simulink model "SimuRun_Day1_Val"  (R2020a)
settings: Solver=FixedStepAuto  StartTime=86400*0+360*60  StopTime=86400*0+1200*60  FixedStep=60  RelTol=1e-6
settings Model: Creator=zhelu  LastModifiedBy=yl3328

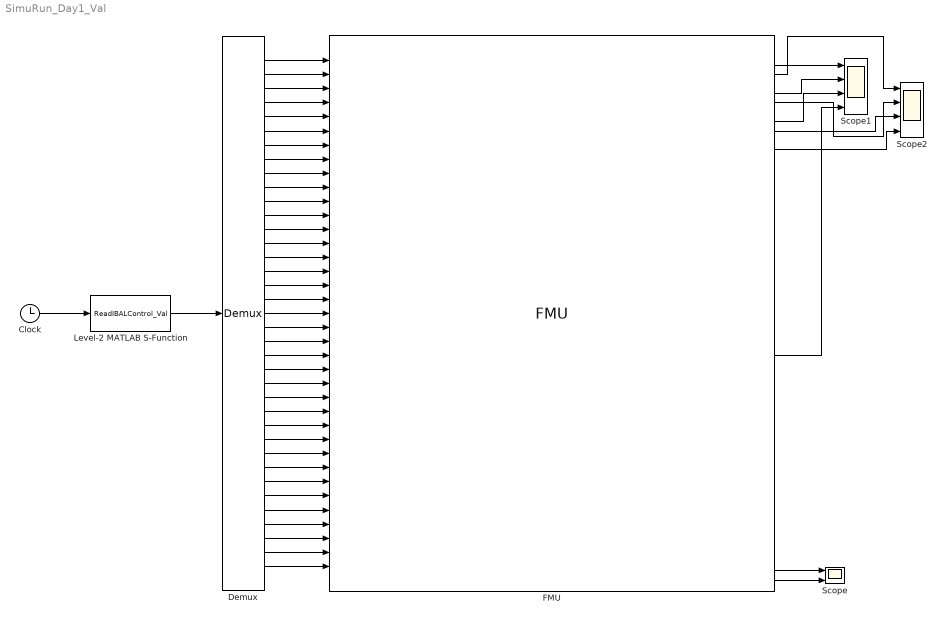
== system SimuRun_Day1_Val ==
  Clock : Clock
  Demux : Demux  Outputs=37
  FMU : FMU  FMUName=All_IBAL_0821.fmu  FMUDebugLogging=on  FMUMode=CoSimulation  FMUIsToleranceUsed=on  FMUToleranceValue=1E-06
      mask Type: All_IBAL_0821 [Co-Simulation, v2.0]
      mask Display:
      | disp('All_IBAL_0821');
      | port_label('output',1,'Power_ahu2_fan');
      | port_label('output',2,'Power_ahu1_fan');
      | port_label('output',3,'m_vav1');
      | port_label('output',4,'T_vav1');
      | port_label('output',5,'w_vav1');
      | port_label('output',6,'m_vav2');
      | port_label('output',7,'T_vav2');
      | port_label('output',8,'w_vav2');
      | port_label('output',9,'m_vav3');
      | port_label('output',10,'T_vav3');
      | port_label('output',11,'w_vav3');
      | port_label('output',12,'T_vav4');
      | port_label('output',13,'w_vav4');
      | port_label('output',14,'m_ahu2_SA');
      | port_label('output',15,'m_ahu2_RA');
      | port_label('output',16,'m_ahu2_EA');
      | port_label('output',17,'m_ahu1_SA');
      | port_label('output',18,'m_ahu1_RA');
      | port_label('output',19,'m_ahu1_EA');
      | port_label('output',20,'T_ahu2_SA');
      | port_label('output',21,'T_ahu2_RA');
      | port_label('output',22,'T_ahu2_EA');
      | port_label('output',23,'T_ahu1_SA');
      | port_label('output',24,'T_ahu1_RA');
      | port_label('output',25,'T_ahu1_EA');
      | port_label('output',26,'T_ahu2coil_ain');
      | port_label('output',27,'T_ahu2coil_aout');
      | port_label('output',28,'w_ahu2coil_ain');
      | port_label('output',29,'w_ahu2coil_aout');
      | port_label('output',30,'T_ahu1coil_ain');
      | port_label('output',31,'w_ahu1coil_ain');
      | port_label('output',32,'T_ahu1coil_aout');
      | port_label('output',33,'w_ahu1coil_aout');
      | port_label('output',34,'m_vav4');
      | port_label('output',35,'Tz_vav1');
      | port_label('output',36,'Tz_vav2');
      | port_label('output',37,'Tz_vav3');
      | port_label('output',38,'Tz_vav4');
      | port_label('output',39,'wz_vav1');
      | port_label('output',40,'wz_vav2');
      | port_label('output',41,'wz_vav3');
      | port_label('output',42,'wz_vav4');
      | port_label('output',43,'Ch1Pump_Power');
      | port_label('output',44,'Ch2Pump_Power');
      | port_label('output',45,'SLPump_Power');
      | port_label('output',46,'Ch1_f');
      | port_label('output',47,'Ch2_f');
      | port_label('output',48,'Bypass_f');
      | port_label('output',49,'HX_f');
      | port_label('output',50,'AHU1_f');
      | port_label('output',51,'AHU2_f');
      | port_label('output',52,'Tw_Ch1_outlet');
      | port_label('output',53,'Tw_Ch2_outlet');
      | port_label('output',54,'Tw_Ch1_inlet');
      | port_label('output',55,'Tw_Ch2_inlet');
      | port_label('output',56,'CondPump_Power');
      | port_label('output',57,'Chiller1_Power');
      | port_label('output',58,'Chiller2_Power');
      | port_label('input',1,'AHU2F');
      | port_label('input',2,'AHU1F');
      | port_label('input',3,'AHU2SAD');
      | port_label('input',4,'AHU2RAD');
      | port_label('input',5,'AHU2EAD');
      | port_label('input',6,'AHU1SAD');
      | port_label('input',7,'AHU1RAD');
      | port_label('input',8,'AHU1EAD');
      | port_label('input',9,'VAV1D');
      | port_label('input',10,'VAV2D');
      | port_label('input',11,'VAV3D');
      | port_label('input',12,'VAV4D');
      | port_label('input',13,'m_ahu2_OA');
      | port_label('input',14,'T_ahu2_OA');
      | port_label('input',15,'w_ahu2_OA');
      | port_label('input',16,'m_ahu1_OA');
      | port_label('input',17,'T_ahu1_OA');
      | port_label('input',18,'w_ahu1_OA');
      | port_label('input',19,'Qs_z1_ahu2');
      | port_label('input',20,'Qs_z2_ahu2');
      | port_label('input',21,'Qs_z1_ahu1');
      | port_label('input',22,'Qs_z2_ahu1');
      | port_label('input',23,'Ql_z1_ahu2');
      | port_label('input',24,'Ql_z2_ahu2');
      | port_label('input',25,'Ql_z1_ahu1');
      | port_label('input',26,'Ql_z2_ahu1');
      | port_label('input',27,'Ch1_status');
      | port_label('input',28,'Ch2_status');
      | port_label('input',29,'Ch1Pump_m');
      | port_label('input',30,'Ch2Pump_m');
      | port_label('input',31,'SLPump_v');
      | port_label('input',32,'AHU1Valve_y');
      | port_label('input',33,'AHU2Valve_y');
      | port_label('input',34,'Teva_out_set_chiller1');
      | port_label('input',35,'Teva_out_set_chiller2');
      | port_label('input',36,'Tw');
      | port_label('input',37,'m_pump_conden');
  Level-2 MATLAB S-Function : M-S-Function  FunctionName=ReadIBALControl_Val
  Scope : Scope  NumInputPorts=2
  Scope1 : Scope  NumInputPorts=4
  Scope2 : Scope  NumInputPorts=4
  wires:
  FMU/57 -> Scope/1
  FMU/58 -> Scope/2
  FMU/3 -> Scope1/1
  FMU/6 -> Scope1/2
  FMU/9 -> Scope1/3
  FMU/34 -> Scope1/4
  FMU/4 -> Scope2/1
  FMU/7 -> Scope2/2
  FMU/10 -> Scope2/3
  FMU/12 -> Scope2/4
  Clock/1 -> Level-2 MATLAB S-Function/1
  Level-2 MATLAB S-Function/1 -> Demux/1
  Demux/1 -> FMU/1
  Demux/2 -> FMU/2
  Demux/3 -> FMU/3
  Demux/4 -> FMU/4
  Demux/5 -> FMU/5
  Demux/6 -> FMU/6
  Demux/7 -> FMU/7
  Demux/8 -> FMU/8
  Demux/9 -> FMU/9
  Demux/10 -> FMU/10
  Demux/11 -> FMU/11
  Demux/12 -> FMU/12
  Demux/13 -> FMU/13
  Demux/14 -> FMU/14
  Demux/15 -> FMU/15
  Demux/16 -> FMU/16
  Demux/17 -> FMU/17
  Demux/18 -> FMU/18
  Demux/19 -> FMU/19
  Demux/20 -> FMU/20
  Demux/21 -> FMU/21
  Demux/22 -> FMU/22
  Demux/23 -> FMU/23
  Demux/24 -> FMU/24
  Demux/25 -> FMU/25
  Demux/26 -> FMU/26
  Demux/27 -> FMU/27
  Demux/28 -> FMU/28
  Demux/29 -> FMU/29
  Demux/30 -> FMU/30
  Demux/31 -> FMU/31
  Demux/32 -> FMU/32
  Demux/33 -> FMU/33
  Demux/34 -> FMU/34
  Demux/35 -> FMU/35
  Demux/36 -> FMU/36
  Demux/37 -> FMU/37
